simulink library "csc_cmp_command_mode_process_mtv_lib"  (R2014b)
settings: Solver=ode45  StartTime=0.0  StopTime=10.0  RelTol=1e-3
undefined symbols (not defined in the file or in its folder): csc_cmp_dt
libraries: util_info_lib x1, csu_cml_command_latch_mtv_lib x1
settings Model: Creator=mstewart  LastModifiedBy=mstewart

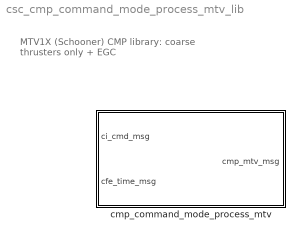
== system csc_cmp_command_mode_process_mtv_lib ==
  note: MTV1X (Schooner) CMP library:
      | coarse thrusters only + EGC
  cmp_command_mode_process_mtv : Subsystem  Tag=OFSW  TreatAsAtomicUnit=on  SystemSampleTime=csc_cmp_dt

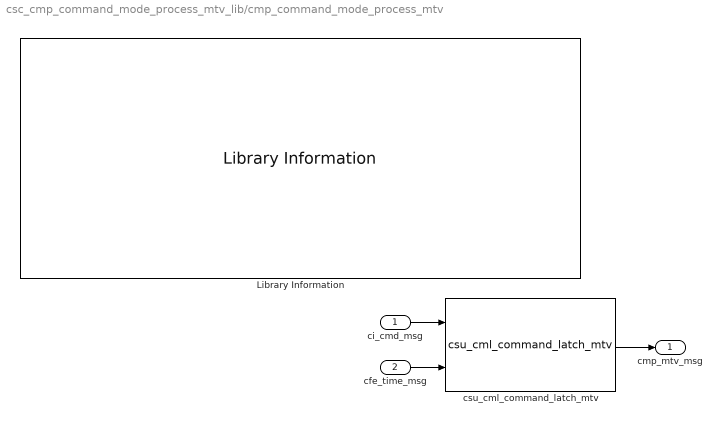
== system csc_cmp_command_mode_process_mtv_lib/cmp_command_mode_process_mtv ==
  ci_cmd_msg : Inport  OutDataTypeStr=Bus: ci_cmd_msg
  cfe_time_msg : Inport  Port=2  OutDataTypeStr=Bus: cfe_time_msg
  Library Information : util_info_lib/Library Information  owner='escrane'
  csu_cml_command_latch_mtv : csu_cml_command_latch_mtv_lib/csu_cml_command_latch_mtv
  cmp_mtv_msg : Outport  OutDataTypeStr=Bus: cmp_mtv_msg
  wires:
  csu_cml_command_latch_mtv/1 -> cmp_mtv_msg/1
  ci_cmd_msg/1 -> csu_cml_command_latch_mtv/1
  cfe_time_msg/1 -> csu_cml_command_latch_mtv/2
